simulink library "MBDS_Subsystems"  (R2018b)
settings: Solver=ode45  StartTime=0.0  StopTime=10.0  RelTol=1e-3
libraries: KIBES_Signal x1429, MBDS_Modules x44, simulink x2
(part 5 of 15)

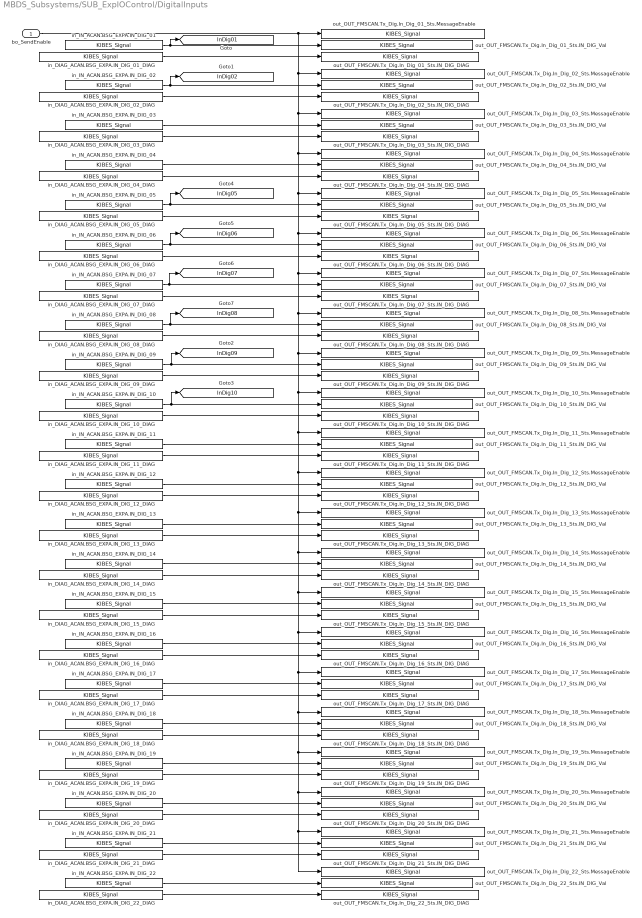
== system MBDS_Subsystems/SUB_ExpIOControl/DigitalInputs ==
  bo_SendEnable : Inport
  in_DIAG_ACAN.BSG_EXPA.IN_DIG_01_DIAG : KIBES_Signal/KIBES_Signal  MBDS_LibraryBlock=on  DatabaseKey=871  SignalName=DIAG_ACAN.BSG_EXPA.IN_DIG_01_DIAG  SymbolName=DIAG_ACAN_BSG_EXPA_IN_DIG_01_DIAG_000871  DataType=uint16  Init=1  Slope=1  Bias=0  DataSize=1  fpDataType=uint16  BlockIOType=Inport  DeviceType=0
  in_DIAG_ACAN.BSG_EXPA.IN_DIG_02_DIAG : KIBES_Signal/KIBES_Signal  MBDS_LibraryBlock=on  DatabaseKey=869  SignalName=DIAG_ACAN.BSG_EXPA.IN_DIG_02_DIAG  SymbolName=DIAG_ACAN_BSG_EXPA_IN_DIG_02_DIAG_000869  DataType=uint16  Init=1  Slope=1  Bias=0  DataSize=1  fpDataType=uint16  BlockIOType=Inport  DeviceType=0
  in_DIAG_ACAN.BSG_EXPA.IN_DIG_03_DIAG : KIBES_Signal/KIBES_Signal  MBDS_LibraryBlock=on  DatabaseKey=867  SignalName=DIAG_ACAN.BSG_EXPA.IN_DIG_03_DIAG  SymbolName=DIAG_ACAN_BSG_EXPA_IN_DIG_03_DIAG_000867  DataType=uint16  Init=1  Slope=1  Bias=0  DataSize=1  fpDataType=uint16  BlockIOType=Inport  DeviceType=0
  in_DIAG_ACAN.BSG_EXPA.IN_DIG_04_DIAG : KIBES_Signal/KIBES_Signal  MBDS_LibraryBlock=on  DatabaseKey=865  SignalName=DIAG_ACAN.BSG_EXPA.IN_DIG_04_DIAG  SymbolName=DIAG_ACAN_BSG_EXPA_IN_DIG_04_DIAG_000865  DataType=uint16  Init=1  Slope=1  Bias=0  DataSize=1  fpDataType=uint16  BlockIOType=Inport  DeviceType=0
  in_DIAG_ACAN.BSG_EXPA.IN_DIG_05_DIAG : KIBES_Signal/KIBES_Signal  MBDS_LibraryBlock=on  DatabaseKey=859  SignalName=DIAG_ACAN.BSG_EXPA.IN_DIG_05_DIAG  SymbolName=DIAG_ACAN_BSG_EXPA_IN_DIG_05_DIAG_000859  DataType=uint16  Init=1  Slope=1  Bias=0  DataSize=1  fpDataType=uint16  BlockIOType=Inport  DeviceType=0
  in_DIAG_ACAN.BSG_EXPA.IN_DIG_06_DIAG : KIBES_Signal/KIBES_Signal  MBDS_LibraryBlock=on  DatabaseKey=862  SignalName=DIAG_ACAN.BSG_EXPA.IN_DIG_06_DIAG  SymbolName=DIAG_ACAN_BSG_EXPA_IN_DIG_06_DIAG_000862  DataType=uint16  Init=1  Slope=1  Bias=0  DataSize=1  fpDataType=uint16  BlockIOType=Inport  DeviceType=0
  in_DIAG_ACAN.BSG_EXPA.IN_DIG_07_DIAG : KIBES_Signal/KIBES_Signal  MBDS_LibraryBlock=on  DatabaseKey=882  SignalName=DIAG_ACAN.BSG_EXPA.IN_DIG_07_DIAG  SymbolName=DIAG_ACAN_BSG_EXPA_IN_DIG_07_DIAG_000882  DataType=uint16  Init=1  Slope=1  Bias=0  DataSize=1  fpDataType=uint16  BlockIOType=Inport  DeviceType=0
  in_DIAG_ACAN.BSG_EXPA.IN_DIG_08_DIAG : KIBES_Signal/KIBES_Signal  MBDS_LibraryBlock=on  DatabaseKey=884  SignalName=DIAG_ACAN.BSG_EXPA.IN_DIG_08_DIAG  SymbolName=DIAG_ACAN_BSG_EXPA_IN_DIG_08_DIAG_000884  DataType=uint16  Init=1  Slope=1  Bias=0  DataSize=1  fpDataType=uint16  BlockIOType=Inport  DeviceType=0
  in_DIAG_ACAN.BSG_EXPA.IN_DIG_09_DIAG : KIBES_Signal/KIBES_Signal  MBDS_LibraryBlock=on  DatabaseKey=880  SignalName=DIAG_ACAN.BSG_EXPA.IN_DIG_09_DIAG  SymbolName=DIAG_ACAN_BSG_EXPA_IN_DIG_09_DIAG_000880  DataType=uint16  Init=1  Slope=1  Bias=0  DataSize=1  fpDataType=uint16  BlockIOType=Inport  DeviceType=0
  in_DIAG_ACAN.BSG_EXPA.IN_DIG_10_DIAG : KIBES_Signal/KIBES_Signal  MBDS_LibraryBlock=on  DatabaseKey=877  SignalName=DIAG_ACAN.BSG_EXPA.IN_DIG_10_DIAG  SymbolName=DIAG_ACAN_BSG_EXPA_IN_DIG_10_DIAG_000877  DataType=uint16  Init=1  Slope=1  Bias=0  DataSize=1  fpDataType=uint16  BlockIOType=Inport  DeviceType=0
  in_DIAG_ACAN.BSG_EXPA.IN_DIG_11_DIAG : KIBES_Signal/KIBES_Signal  MBDS_LibraryBlock=on  DatabaseKey=849  SignalName=DIAG_ACAN.BSG_EXPA.IN_DIG_11_DIAG  SymbolName=DIAG_ACAN_BSG_EXPA_IN_DIG_11_DIAG_000849  DataType=uint16  Init=1  Slope=1  Bias=0  DataSize=1  fpDataType=uint16  BlockIOType=Inport  DeviceType=0
  in_DIAG_ACAN.BSG_EXPA.IN_DIG_12_DIAG : KIBES_Signal/KIBES_Signal  MBDS_LibraryBlock=on  DatabaseKey=841  SignalName=DIAG_ACAN.BSG_EXPA.IN_DIG_12_DIAG  SymbolName=DIAG_ACAN_BSG_EXPA_IN_DIG_12_DIAG_000841  DataType=uint16  Init=1  Slope=1  Bias=0  DataSize=1  fpDataType=uint16  BlockIOType=Inport  DeviceType=0
  in_DIAG_ACAN.BSG_EXPA.IN_DIG_13_DIAG : KIBES_Signal/KIBES_Signal  MBDS_LibraryBlock=on  DatabaseKey=843  SignalName=DIAG_ACAN.BSG_EXPA.IN_DIG_13_DIAG  SymbolName=DIAG_ACAN_BSG_EXPA_IN_DIG_13_DIAG_000843  DataType=uint16  Init=1  Slope=1  Bias=0  DataSize=1  fpDataType=uint16  BlockIOType=Inport  DeviceType=0
  in_DIAG_ACAN.BSG_EXPA.IN_DIG_14_DIAG : KIBES_Signal/KIBES_Signal  MBDS_LibraryBlock=on  DatabaseKey=857  SignalName=DIAG_ACAN.BSG_EXPA.IN_DIG_14_DIAG  SymbolName=DIAG_ACAN_BSG_EXPA_IN_DIG_14_DIAG_000857  DataType=uint16  Init=1  Slope=1  Bias=0  DataSize=1  fpDataType=uint16  BlockIOType=Inport  DeviceType=0
  in_DIAG_ACAN.BSG_EXPA.IN_DIG_15_DIAG : KIBES_Signal/KIBES_Signal  MBDS_LibraryBlock=on  DatabaseKey=855  SignalName=DIAG_ACAN.BSG_EXPA.IN_DIG_15_DIAG  SymbolName=DIAG_ACAN_BSG_EXPA_IN_DIG_15_DIAG_000855  DataType=uint16  Init=1  Slope=1  Bias=0  DataSize=1  fpDataType=uint16  BlockIOType=Inport  DeviceType=0
  in_DIAG_ACAN.BSG_EXPA.IN_DIG_16_DIAG : KIBES_Signal/KIBES_Signal  MBDS_LibraryBlock=on  DatabaseKey=847  SignalName=DIAG_ACAN.BSG_EXPA.IN_DIG_16_DIAG  SymbolName=DIAG_ACAN_BSG_EXPA_IN_DIG_16_DIAG_000847  DataType=uint16  Init=1  Slope=1  Bias=0  DataSize=1  fpDataType=uint16  BlockIOType=Inport  DeviceType=0
  in_DIAG_ACAN.BSG_EXPA.IN_DIG_17_DIAG : KIBES_Signal/KIBES_Signal  MBDS_LibraryBlock=on  DatabaseKey=861  SignalName=DIAG_ACAN.BSG_EXPA.IN_DIG_17_DIAG  SymbolName=DIAG_ACAN_BSG_EXPA_IN_DIG_17_DIAG_000861  DataType=uint16  Init=1  Slope=1  Bias=0  DataSize=1  fpDataType=uint16  BlockIOType=Inport  DeviceType=0
  in_DIAG_ACAN.BSG_EXPA.IN_DIG_18_DIAG : KIBES_Signal/KIBES_Signal  MBDS_LibraryBlock=on  DatabaseKey=851  SignalName=DIAG_ACAN.BSG_EXPA.IN_DIG_18_DIAG  SymbolName=DIAG_ACAN_BSG_EXPA_IN_DIG_18_DIAG_000851  DataType=uint16  Init=1  Slope=1  Bias=0  DataSize=1  fpDataType=uint16  BlockIOType=Inport  DeviceType=0
  in_DIAG_ACAN.BSG_EXPA.IN_DIG_19_DIAG : KIBES_Signal/KIBES_Signal  MBDS_LibraryBlock=on  DatabaseKey=842  SignalName=DIAG_ACAN.BSG_EXPA.IN_DIG_19_DIAG  SymbolName=DIAG_ACAN_BSG_EXPA_IN_DIG_19_DIAG_000842  DataType=uint16  Init=1  Slope=1  Bias=0  DataSize=1  fpDataType=uint16  BlockIOType=Inport  DeviceType=0
  in_DIAG_ACAN.BSG_EXPA.IN_DIG_20_DIAG : KIBES_Signal/KIBES_Signal  MBDS_LibraryBlock=on  DatabaseKey=846  SignalName=DIAG_ACAN.BSG_EXPA.IN_DIG_20_DIAG  SymbolName=DIAG_ACAN_BSG_EXPA_IN_DIG_20_DIAG_000846  DataType=uint16  Init=1  Slope=1  Bias=0  DataSize=1  fpDataType=uint16  BlockIOType=Inport  DeviceType=0
  in_DIAG_ACAN.BSG_EXPA.IN_DIG_21_DIAG : KIBES_Signal/KIBES_Signal  MBDS_LibraryBlock=on  DatabaseKey=875  SignalName=DIAG_ACAN.BSG_EXPA.IN_DIG_21_DIAG  SymbolName=DIAG_ACAN_BSG_EXPA_IN_DIG_21_DIAG_000875  DataType=uint16  Init=1  Slope=1  Bias=0  DataSize=1  fpDataType=uint16  BlockIOType=Inport  DeviceType=0
  in_DIAG_ACAN.BSG_EXPA.IN_DIG_22_DIAG : KIBES_Signal/KIBES_Signal  MBDS_LibraryBlock=on  DatabaseKey=873  SignalName=DIAG_ACAN.BSG_EXPA.IN_DIG_22_DIAG  SymbolName=DIAG_ACAN_BSG_EXPA_IN_DIG_22_DIAG_000873  DataType=uint16  Init=1  Slope=1  Bias=0  DataSize=1  fpDataType=uint16  BlockIOType=Inport  DeviceType=0
  in_IN_ACAN.BSG_EXPA.IN_DIG_01 : KIBES_Signal/KIBES_Signal  MBDS_LibraryBlock=on  DatabaseKey=872  SignalName=IN_ACAN.BSG_EXPA.IN_DIG_01  SymbolName=IN_ACAN_BSG_EXPA_IN_DIG_01_000872  DataType=boolean  Init=0  Slope=1  Bias=0  DataSize=1  fpDataType=boolean  BlockIOType=Inport  DeviceType=0
  in_IN_ACAN.BSG_EXPA.IN_DIG_02 : KIBES_Signal/KIBES_Signal  MBDS_LibraryBlock=on  DatabaseKey=878  SignalName=IN_ACAN.BSG_EXPA.IN_DIG_02  SymbolName=IN_ACAN_BSG_EXPA_IN_DIG_02_000878  DataType=boolean  Init=0  Slope=1  Bias=0  DataSize=1  fpDataType=boolean  BlockIOType=Inport  DeviceType=0
  in_IN_ACAN.BSG_EXPA.IN_DIG_03 : KIBES_Signal/KIBES_Signal  MBDS_LibraryBlock=on  DatabaseKey=870  SignalName=IN_ACAN.BSG_EXPA.IN_DIG_03  SymbolName=IN_ACAN_BSG_EXPA_IN_DIG_03_000870  DataType=boolean  Init=0  Slope=1  Bias=0  DataSize=1  fpDataType=boolean  BlockIOType=Inport  DeviceType=0
  in_IN_ACAN.BSG_EXPA.IN_DIG_04 : KIBES_Signal/KIBES_Signal  MBDS_LibraryBlock=on  DatabaseKey=866  SignalName=IN_ACAN.BSG_EXPA.IN_DIG_04  SymbolName=IN_ACAN_BSG_EXPA_IN_DIG_04_000866  DataType=boolean  Init=0  Slope=1  Bias=0  DataSize=1  fpDataType=boolean  BlockIOType=Inport  DeviceType=0
  in_IN_ACAN.BSG_EXPA.IN_DIG_05 : KIBES_Signal/KIBES_Signal  MBDS_LibraryBlock=on  DatabaseKey=864  SignalName=IN_ACAN.BSG_EXPA.IN_DIG_05  SymbolName=IN_ACAN_BSG_EXPA_IN_DIG_05_000864  DataType=boolean  Init=0  Slope=1  Bias=0  DataSize=1  fpDataType=boolean  BlockIOType=Inport  DeviceType=0
  in_IN_ACAN.BSG_EXPA.IN_DIG_06 : KIBES_Signal/KIBES_Signal  MBDS_LibraryBlock=on  DatabaseKey=863  SignalName=IN_ACAN.BSG_EXPA.IN_DIG_06  SymbolName=IN_ACAN_BSG_EXPA_IN_DIG_06_000863  DataType=boolean  Init=0  Slope=1  Bias=0  DataSize=1  fpDataType=boolean  BlockIOType=Inport  DeviceType=0
  in_IN_ACAN.BSG_EXPA.IN_DIG_07 : KIBES_Signal/KIBES_Signal  MBDS_LibraryBlock=on  DatabaseKey=868  SignalName=IN_ACAN.BSG_EXPA.IN_DIG_07  SymbolName=IN_ACAN_BSG_EXPA_IN_DIG_07_000868  DataType=boolean  Init=0  Slope=1  Bias=0  DataSize=1  fpDataType=boolean  BlockIOType=Inport  DeviceType=0
  in_IN_ACAN.BSG_EXPA.IN_DIG_08 : KIBES_Signal/KIBES_Signal  MBDS_LibraryBlock=on  DatabaseKey=883  SignalName=IN_ACAN.BSG_EXPA.IN_DIG_08  SymbolName=IN_ACAN_BSG_EXPA_IN_DIG_08_000883  DataType=boolean  Init=0  Slope=1  Bias=0  DataSize=1  fpDataType=boolean  BlockIOType=Inport  DeviceType=0
  in_IN_ACAN.BSG_EXPA.IN_DIG_09 : KIBES_Signal/KIBES_Signal  MBDS_LibraryBlock=on  DatabaseKey=881  SignalName=IN_ACAN.BSG_EXPA.IN_DIG_09  SymbolName=IN_ACAN_BSG_EXPA_IN_DIG_09_000881  DataType=boolean  Init=0  Slope=1  Bias=0  DataSize=1  fpDataType=boolean  BlockIOType=Inport  DeviceType=0
  in_IN_ACAN.BSG_EXPA.IN_DIG_10 : KIBES_Signal/KIBES_Signal  MBDS_LibraryBlock=on  DatabaseKey=879  SignalName=IN_ACAN.BSG_EXPA.IN_DIG_10  SymbolName=IN_ACAN_BSG_EXPA_IN_DIG_10_000879  DataType=boolean  Init=0  Slope=1  Bias=0  DataSize=1  fpDataType=boolean  BlockIOType=Inport  DeviceType=0
  in_IN_ACAN.BSG_EXPA.IN_DIG_11 : KIBES_Signal/KIBES_Signal  MBDS_LibraryBlock=on  DatabaseKey=860  SignalName=IN_ACAN.BSG_EXPA.IN_DIG_11  SymbolName=IN_ACAN_BSG_EXPA_IN_DIG_11_000860  DataType=boolean  Init=0  Slope=1  Bias=0  DataSize=1  fpDataType=boolean  BlockIOType=Inport  DeviceType=0
  in_IN_ACAN.BSG_EXPA.IN_DIG_12 : KIBES_Signal/KIBES_Signal  MBDS_LibraryBlock=on  DatabaseKey=848  SignalName=IN_ACAN.BSG_EXPA.IN_DIG_12  SymbolName=IN_ACAN_BSG_EXPA_IN_DIG_12_000848  DataType=boolean  Init=0  Slope=1  Bias=0  DataSize=1  fpDataType=boolean  BlockIOType=Inport  DeviceType=0
  in_IN_ACAN.BSG_EXPA.IN_DIG_13 : KIBES_Signal/KIBES_Signal  MBDS_LibraryBlock=on  DatabaseKey=844  SignalName=IN_ACAN.BSG_EXPA.IN_DIG_13  SymbolName=IN_ACAN_BSG_EXPA_IN_DIG_13_000844  DataType=boolean  Init=0  Slope=1  Bias=0  DataSize=1  fpDataType=boolean  BlockIOType=Inport  DeviceType=0
  in_IN_ACAN.BSG_EXPA.IN_DIG_14 : KIBES_Signal/KIBES_Signal  MBDS_LibraryBlock=on  DatabaseKey=858  SignalName=IN_ACAN.BSG_EXPA.IN_DIG_14  SymbolName=IN_ACAN_BSG_EXPA_IN_DIG_14_000858  DataType=boolean  Init=0  Slope=1  Bias=0  DataSize=1  fpDataType=boolean  BlockIOType=Inport  DeviceType=0
  in_IN_ACAN.BSG_EXPA.IN_DIG_15 : KIBES_Signal/KIBES_Signal  MBDS_LibraryBlock=on  DatabaseKey=856  SignalName=IN_ACAN.BSG_EXPA.IN_DIG_15  SymbolName=IN_ACAN_BSG_EXPA_IN_DIG_15_000856  DataType=boolean  Init=0  Slope=1  Bias=0  DataSize=1  fpDataType=boolean  BlockIOType=Inport  DeviceType=0
  in_IN_ACAN.BSG_EXPA.IN_DIG_16 : KIBES_Signal/KIBES_Signal  MBDS_LibraryBlock=on  DatabaseKey=854  SignalName=IN_ACAN.BSG_EXPA.IN_DIG_16  SymbolName=IN_ACAN_BSG_EXPA_IN_DIG_16_000854  DataType=boolean  Init=0  Slope=1  Bias=0  DataSize=1  fpDataType=boolean  BlockIOType=Inport  DeviceType=0
  in_IN_ACAN.BSG_EXPA.IN_DIG_17 : KIBES_Signal/KIBES_Signal  MBDS_LibraryBlock=on  DatabaseKey=853  SignalName=IN_ACAN.BSG_EXPA.IN_DIG_17  SymbolName=IN_ACAN_BSG_EXPA_IN_DIG_17_000853  DataType=boolean  Init=0  Slope=1  Bias=0  DataSize=1  fpDataType=boolean  BlockIOType=Inport  DeviceType=0
  in_IN_ACAN.BSG_EXPA.IN_DIG_18 : KIBES_Signal/KIBES_Signal  MBDS_LibraryBlock=on  DatabaseKey=852  SignalName=IN_ACAN.BSG_EXPA.IN_DIG_18  SymbolName=IN_ACAN_BSG_EXPA_IN_DIG_18_000852  DataType=boolean  Init=0  Slope=1  Bias=0  DataSize=1  fpDataType=boolean  BlockIOType=Inport  DeviceType=0
  in_IN_ACAN.BSG_EXPA.IN_DIG_19 : KIBES_Signal/KIBES_Signal  MBDS_LibraryBlock=on  DatabaseKey=845  SignalName=IN_ACAN.BSG_EXPA.IN_DIG_19  SymbolName=IN_ACAN_BSG_EXPA_IN_DIG_19_000845  DataType=boolean  Init=0  Slope=1  Bias=0  DataSize=1  fpDataType=boolean  BlockIOType=Inport  DeviceType=0
  in_IN_ACAN.BSG_EXPA.IN_DIG_20 : KIBES_Signal/KIBES_Signal  MBDS_LibraryBlock=on  DatabaseKey=850  SignalName=IN_ACAN.BSG_EXPA.IN_DIG_20  SymbolName=IN_ACAN_BSG_EXPA_IN_DIG_20_000850  DataType=boolean  Init=0  Slope=1  Bias=0  DataSize=1  fpDataType=boolean  BlockIOType=Inport  DeviceType=0
  in_IN_ACAN.BSG_EXPA.IN_DIG_21 : KIBES_Signal/KIBES_Signal  MBDS_LibraryBlock=on  DatabaseKey=876  SignalName=IN_ACAN.BSG_EXPA.IN_DIG_21  SymbolName=IN_ACAN_BSG_EXPA_IN_DIG_21_000876  DataType=boolean  Init=0  Slope=1  Bias=0  DataSize=1  fpDataType=boolean  BlockIOType=Inport  DeviceType=0
  in_IN_ACAN.BSG_EXPA.IN_DIG_22 : KIBES_Signal/KIBES_Signal  MBDS_LibraryBlock=on  DatabaseKey=874  SignalName=IN_ACAN.BSG_EXPA.IN_DIG_22  SymbolName=IN_ACAN_BSG_EXPA_IN_DIG_22_000874  DataType=boolean  Init=0  Slope=1  Bias=0  DataSize=1  fpDataType=boolean  BlockIOType=Inport  DeviceType=0
  out_OUT_FMSCAN.Tx_Dig.In_Dig_01_Sts.IN_DIG_DIAG : KIBES_Signal/KIBES_Signal  MBDS_LibraryBlock=on  DatabaseKey=2366  SignalName=OUT_FMSCAN.Tx_Dig.In_Dig_01_Sts.IN_DIG_DIAG  SymbolName=OUT_FMSCAN_Tx_Dig_In_Dig_01_Sts_IN_DIG_DIAG_002366  DataType=uint16  Init=0  Slope=1  Bias=0  DataSize=1  fpDataType=uint16  BlockIOType=Outport  DeviceType=0
  out_OUT_FMSCAN.Tx_Dig.In_Dig_01_Sts.IN_DIG_Val : KIBES_Signal/KIBES_Signal  MBDS_LibraryBlock=on  DatabaseKey=2367  SignalName=OUT_FMSCAN.Tx_Dig.In_Dig_01_Sts.IN_DIG_Val  SymbolName=OUT_FMSCAN_Tx_Dig_In_Dig_01_Sts_IN_DIG_Val_002367  DataType=boolean  Init=0  Slope=1  Bias=0  DataSize=1  fpDataType=boolean  BlockIOType=Outport  DeviceType=0
  out_OUT_FMSCAN.Tx_Dig.In_Dig_01_Sts.MessageEnable : KIBES_Signal/KIBES_Signal  MBDS_LibraryBlock=on  DatabaseKey=2410  SignalName=OUT_FMSCAN.Tx_Dig.In_Dig_01_Sts.MessageEnable  SymbolName=OUT_FMSCAN_Tx_Dig_In_Dig_01_Sts_MessageEnable_002410  DataType=boolean  Init=0  Slope=1  Bias=0  DataSize=1  fpDataType=boolean  BlockIOType=Outport  DeviceType=0
  out_OUT_FMSCAN.Tx_Dig.In_Dig_02_Sts.IN_DIG_DIAG : KIBES_Signal/KIBES_Signal  MBDS_LibraryBlock=on  DatabaseKey=2368  SignalName=OUT_FMSCAN.Tx_Dig.In_Dig_02_Sts.IN_DIG_DIAG  SymbolName=OUT_FMSCAN_Tx_Dig_In_Dig_02_Sts_IN_DIG_DIAG_002368  DataType=uint16  Init=0  Slope=1  Bias=0  DataSize=1  fpDataType=uint16  BlockIOType=Outport  DeviceType=0
  out_OUT_FMSCAN.Tx_Dig.In_Dig_02_Sts.IN_DIG_Val : KIBES_Signal/KIBES_Signal  MBDS_LibraryBlock=on  DatabaseKey=2369  SignalName=OUT_FMSCAN.Tx_Dig.In_Dig_02_Sts.IN_DIG_Val  SymbolName=OUT_FMSCAN_Tx_Dig_In_Dig_02_Sts_IN_DIG_Val_002369  DataType=boolean  Init=0  Slope=1  Bias=0  DataSize=1  fpDataType=boolean  BlockIOType=Outport  DeviceType=0
  out_OUT_FMSCAN.Tx_Dig.In_Dig_02_Sts.MessageEnable : KIBES_Signal/KIBES_Signal  MBDS_LibraryBlock=on  DatabaseKey=2411  SignalName=OUT_FMSCAN.Tx_Dig.In_Dig_02_Sts.MessageEnable  SymbolName=OUT_FMSCAN_Tx_Dig_In_Dig_02_Sts_MessageEnable_002411  DataType=boolean  Init=0  Slope=1  Bias=0  DataSize=1  fpDataType=boolean  BlockIOType=Outport  DeviceType=0
  out_OUT_FMSCAN.Tx_Dig.In_Dig_03_Sts.IN_DIG_DIAG : KIBES_Signal/KIBES_Signal  MBDS_LibraryBlock=on  DatabaseKey=2370  SignalName=OUT_FMSCAN.Tx_Dig.In_Dig_03_Sts.IN_DIG_DIAG  SymbolName=OUT_FMSCAN_Tx_Dig_In_Dig_03_Sts_IN_DIG_DIAG_002370  DataType=uint16  Init=0  Slope=1  Bias=0  DataSize=1  fpDataType=uint16  BlockIOType=Outport  DeviceType=0
  out_OUT_FMSCAN.Tx_Dig.In_Dig_03_Sts.IN_DIG_Val : KIBES_Signal/KIBES_Signal  MBDS_LibraryBlock=on  DatabaseKey=2371  SignalName=OUT_FMSCAN.Tx_Dig.In_Dig_03_Sts.IN_DIG_Val  SymbolName=OUT_FMSCAN_Tx_Dig_In_Dig_03_Sts_IN_DIG_Val_002371  DataType=boolean  Init=0  Slope=1  Bias=0  DataSize=1  fpDataType=boolean  BlockIOType=Outport  DeviceType=0
  out_OUT_FMSCAN.Tx_Dig.In_Dig_03_Sts.MessageEnable : KIBES_Signal/KIBES_Signal  MBDS_LibraryBlock=on  DatabaseKey=2412  SignalName=OUT_FMSCAN.Tx_Dig.In_Dig_03_Sts.MessageEnable  SymbolName=OUT_FMSCAN_Tx_Dig_In_Dig_03_Sts_MessageEnable_002412  DataType=boolean  Init=0  Slope=1  Bias=0  DataSize=1  fpDataType=boolean  BlockIOType=Outport  DeviceType=0
  out_OUT_FMSCAN.Tx_Dig.In_Dig_04_Sts.IN_DIG_DIAG : KIBES_Signal/KIBES_Signal  MBDS_LibraryBlock=on  DatabaseKey=2372  SignalName=OUT_FMSCAN.Tx_Dig.In_Dig_04_Sts.IN_DIG_DIAG  SymbolName=OUT_FMSCAN_Tx_Dig_In_Dig_04_Sts_IN_DIG_DIAG_002372  DataType=uint16  Init=0  Slope=1  Bias=0  DataSize=1  fpDataType=uint16  BlockIOType=Outport  DeviceType=0
  out_OUT_FMSCAN.Tx_Dig.In_Dig_04_Sts.IN_DIG_Val : KIBES_Signal/KIBES_Signal  MBDS_LibraryBlock=on  DatabaseKey=2373  SignalName=OUT_FMSCAN.Tx_Dig.In_Dig_04_Sts.IN_DIG_Val  SymbolName=OUT_FMSCAN_Tx_Dig_In_Dig_04_Sts_IN_DIG_Val_002373  DataType=boolean  Init=0  Slope=1  Bias=0  DataSize=1  fpDataType=boolean  BlockIOType=Outport  DeviceType=0
  out_OUT_FMSCAN.Tx_Dig.In_Dig_04_Sts.MessageEnable : KIBES_Signal/KIBES_Signal  MBDS_LibraryBlock=on  DatabaseKey=2413  SignalName=OUT_FMSCAN.Tx_Dig.In_Dig_04_Sts.MessageEnable  SymbolName=OUT_FMSCAN_Tx_Dig_In_Dig_04_Sts_MessageEnable_002413  DataType=boolean  Init=0  Slope=1  Bias=0  DataSize=1  fpDataType=boolean  BlockIOType=Outport  DeviceType=0
  out_OUT_FMSCAN.Tx_Dig.In_Dig_05_Sts.IN_DIG_DIAG : KIBES_Signal/KIBES_Signal  MBDS_LibraryBlock=on  DatabaseKey=2374  SignalName=OUT_FMSCAN.Tx_Dig.In_Dig_05_Sts.IN_DIG_DIAG  SymbolName=OUT_FMSCAN_Tx_Dig_In_Dig_05_Sts_IN_DIG_DIAG_002374  DataType=uint16  Init=0  Slope=1  Bias=0  DataSize=1  fpDataType=uint16  BlockIOType=Outport  DeviceType=0
  out_OUT_FMSCAN.Tx_Dig.In_Dig_05_Sts.IN_DIG_Val : KIBES_Signal/KIBES_Signal  MBDS_LibraryBlock=on  DatabaseKey=2375  SignalName=OUT_FMSCAN.Tx_Dig.In_Dig_05_Sts.IN_DIG_Val  SymbolName=OUT_FMSCAN_Tx_Dig_In_Dig_05_Sts_IN_DIG_Val_002375  DataType=boolean  Init=0  Slope=1  Bias=0  DataSize=1  fpDataType=boolean  BlockIOType=Outport  DeviceType=0
  out_OUT_FMSCAN.Tx_Dig.In_Dig_05_Sts.MessageEnable : KIBES_Signal/KIBES_Signal  MBDS_LibraryBlock=on  DatabaseKey=2414  SignalName=OUT_FMSCAN.Tx_Dig.In_Dig_05_Sts.MessageEnable  SymbolName=OUT_FMSCAN_Tx_Dig_In_Dig_05_Sts_MessageEnable_002414  DataType=boolean  Init=0  Slope=1  Bias=0  DataSize=1  fpDataType=boolean  BlockIOType=Outport  DeviceType=0
  out_OUT_FMSCAN.Tx_Dig.In_Dig_06_Sts.IN_DIG_DIAG : KIBES_Signal/KIBES_Signal  MBDS_LibraryBlock=on  DatabaseKey=2376  SignalName=OUT_FMSCAN.Tx_Dig.In_Dig_06_Sts.IN_DIG_DIAG  SymbolName=OUT_FMSCAN_Tx_Dig_In_Dig_06_Sts_IN_DIG_DIAG_002376  DataType=uint16  Init=0  Slope=1  Bias=0  DataSize=1  fpDataType=uint16  BlockIOType=Outport  DeviceType=0
  out_OUT_FMSCAN.Tx_Dig.In_Dig_06_Sts.IN_DIG_Val : KIBES_Signal/KIBES_Signal  MBDS_LibraryBlock=on  DatabaseKey=2377  SignalName=OUT_FMSCAN.Tx_Dig.In_Dig_06_Sts.IN_DIG_Val  SymbolName=OUT_FMSCAN_Tx_Dig_In_Dig_06_Sts_IN_DIG_Val_002377  DataType=boolean  Init=0  Slope=1  Bias=0  DataSize=1  fpDataType=boolean  BlockIOType=Outport  DeviceType=0
  out_OUT_FMSCAN.Tx_Dig.In_Dig_06_Sts.MessageEnable : KIBES_Signal/KIBES_Signal  MBDS_LibraryBlock=on  DatabaseKey=2415  SignalName=OUT_FMSCAN.Tx_Dig.In_Dig_06_Sts.MessageEnable  SymbolName=OUT_FMSCAN_Tx_Dig_In_Dig_06_Sts_MessageEnable_002415  DataType=boolean  Init=0  Slope=1  Bias=0  DataSize=1  fpDataType=boolean  BlockIOType=Outport  DeviceType=0
  out_OUT_FMSCAN.Tx_Dig.In_Dig_07_Sts.IN_DIG_DIAG : KIBES_Signal/KIBES_Signal  MBDS_LibraryBlock=on  DatabaseKey=2378  SignalName=OUT_FMSCAN.Tx_Dig.In_Dig_07_Sts.IN_DIG_DIAG  SymbolName=OUT_FMSCAN_Tx_Dig_In_Dig_07_Sts_IN_DIG_DIAG_002378  DataType=uint16  Init=0  Slope=1  Bias=0  DataSize=1  fpDataType=uint16  BlockIOType=Outport  DeviceType=0
  out_OUT_FMSCAN.Tx_Dig.In_Dig_07_Sts.IN_DIG_Val : KIBES_Signal/KIBES_Signal  MBDS_LibraryBlock=on  DatabaseKey=2379  SignalName=OUT_FMSCAN.Tx_Dig.In_Dig_07_Sts.IN_DIG_Val  SymbolName=OUT_FMSCAN_Tx_Dig_In_Dig_07_Sts_IN_DIG_Val_002379  DataType=boolean  Init=0  Slope=1  Bias=0  DataSize=1  fpDataType=boolean  BlockIOType=Outport  DeviceType=0
  out_OUT_FMSCAN.Tx_Dig.In_Dig_07_Sts.MessageEnable : KIBES_Signal/KIBES_Signal  MBDS_LibraryBlock=on  DatabaseKey=2416  SignalName=OUT_FMSCAN.Tx_Dig.In_Dig_07_Sts.MessageEnable  SymbolName=OUT_FMSCAN_Tx_Dig_In_Dig_07_Sts_MessageEnable_002416  DataType=boolean  Init=0  Slope=1  Bias=0  DataSize=1  fpDataType=boolean  BlockIOType=Outport  DeviceType=0
  out_OUT_FMSCAN.Tx_Dig.In_Dig_08_Sts.IN_DIG_DIAG : KIBES_Signal/KIBES_Signal  MBDS_LibraryBlock=on  DatabaseKey=2380  SignalName=OUT_FMSCAN.Tx_Dig.In_Dig_08_Sts.IN_DIG_DIAG  SymbolName=OUT_FMSCAN_Tx_Dig_In_Dig_08_Sts_IN_DIG_DIAG_002380  DataType=uint16  Init=0  Slope=1  Bias=0  DataSize=1  fpDataType=uint16  BlockIOType=Outport  DeviceType=0
  out_OUT_FMSCAN.Tx_Dig.In_Dig_08_Sts.IN_DIG_Val : KIBES_Signal/KIBES_Signal  MBDS_LibraryBlock=on  DatabaseKey=2381  SignalName=OUT_FMSCAN.Tx_Dig.In_Dig_08_Sts.IN_DIG_Val  SymbolName=OUT_FMSCAN_Tx_Dig_In_Dig_08_Sts_IN_DIG_Val_002381  DataType=boolean  Init=0  Slope=1  Bias=0  DataSize=1  fpDataType=boolean  BlockIOType=Outport  DeviceType=0
  out_OUT_FMSCAN.Tx_Dig.In_Dig_08_Sts.MessageEnable : KIBES_Signal/KIBES_Signal  MBDS_LibraryBlock=on  DatabaseKey=2417  SignalName=OUT_FMSCAN.Tx_Dig.In_Dig_08_Sts.MessageEnable  SymbolName=OUT_FMSCAN_Tx_Dig_In_Dig_08_Sts_MessageEnable_002417  DataType=boolean  Init=0  Slope=1  Bias=0  DataSize=1  fpDataType=boolean  BlockIOType=Outport  DeviceType=0
  out_OUT_FMSCAN.Tx_Dig.In_Dig_09_Sts.IN_DIG_DIAG : KIBES_Signal/KIBES_Signal  MBDS_LibraryBlock=on  DatabaseKey=2382  SignalName=OUT_FMSCAN.Tx_Dig.In_Dig_09_Sts.IN_DIG_DIAG  SymbolName=OUT_FMSCAN_Tx_Dig_In_Dig_09_Sts_IN_DIG_DIAG_002382  DataType=uint16  Init=0  Slope=1  Bias=0  DataSize=1  fpDataType=uint16  BlockIOType=Outport  DeviceType=0
  out_OUT_FMSCAN.Tx_Dig.In_Dig_09_Sts.IN_DIG_Val : KIBES_Signal/KIBES_Signal  MBDS_LibraryBlock=on  DatabaseKey=2383  SignalName=OUT_FMSCAN.Tx_Dig.In_Dig_09_Sts.IN_DIG_Val  SymbolName=OUT_FMSCAN_Tx_Dig_In_Dig_09_Sts_IN_DIG_Val_002383  DataType=boolean  Init=0  Slope=1  Bias=0  DataSize=1  fpDataType=boolean  BlockIOType=Outport  DeviceType=0
  out_OUT_FMSCAN.Tx_Dig.In_Dig_09_Sts.MessageEnable : KIBES_Signal/KIBES_Signal  MBDS_LibraryBlock=on  DatabaseKey=2418  SignalName=OUT_FMSCAN.Tx_Dig.In_Dig_09_Sts.MessageEnable  SymbolName=OUT_FMSCAN_Tx_Dig_In_Dig_09_Sts_MessageEnable_002418  DataType=boolean  Init=0  Slope=1  Bias=0  DataSize=1  fpDataType=boolean  BlockIOType=Outport  DeviceType=0
  out_OUT_FMSCAN.Tx_Dig.In_Dig_10_Sts.IN_DIG_DIAG : KIBES_Signal/KIBES_Signal  MBDS_LibraryBlock=on  DatabaseKey=2384  SignalName=OUT_FMSCAN.Tx_Dig.In_Dig_10_Sts.IN_DIG_DIAG  SymbolName=OUT_FMSCAN_Tx_Dig_In_Dig_10_Sts_IN_DIG_DIAG_002384  DataType=uint16  Init=0  Slope=1  Bias=0  DataSize=1  fpDataType=uint16  BlockIOType=Outport  DeviceType=0
  out_OUT_FMSCAN.Tx_Dig.In_Dig_10_Sts.IN_DIG_Val : KIBES_Signal/KIBES_Signal  MBDS_LibraryBlock=on  DatabaseKey=2385  SignalName=OUT_FMSCAN.Tx_Dig.In_Dig_10_Sts.IN_DIG_Val  SymbolName=OUT_FMSCAN_Tx_Dig_In_Dig_10_Sts_IN_DIG_Val_002385  DataType=boolean  Init=0  Slope=1  Bias=0  DataSize=1  fpDataType=boolean  BlockIOType=Outport  DeviceType=0
  out_OUT_FMSCAN.Tx_Dig.In_Dig_10_Sts.MessageEnable : KIBES_Signal/KIBES_Signal  MBDS_LibraryBlock=on  DatabaseKey=2419  SignalName=OUT_FMSCAN.Tx_Dig.In_Dig_10_Sts.MessageEnable  SymbolName=OUT_FMSCAN_Tx_Dig_In_Dig_10_Sts_MessageEnable_002419  DataType=boolean  Init=0  Slope=1  Bias=0  DataSize=1  fpDataType=boolean  BlockIOType=Outport  DeviceType=0
  out_OUT_FMSCAN.Tx_Dig.In_Dig_11_Sts.IN_DIG_DIAG : KIBES_Signal/KIBES_Signal  MBDS_LibraryBlock=on  DatabaseKey=2386  SignalName=OUT_FMSCAN.Tx_Dig.In_Dig_11_Sts.IN_DIG_DIAG  SymbolName=OUT_FMSCAN_Tx_Dig_In_Dig_11_Sts_IN_DIG_DIAG_002386  DataType=uint16  Init=0  Slope=1  Bias=0  DataSize=1  fpDataType=uint16  BlockIOType=Outport  DeviceType=0
  out_OUT_FMSCAN.Tx_Dig.In_Dig_11_Sts.IN_DIG_Val : KIBES_Signal/KIBES_Signal  MBDS_LibraryBlock=on  DatabaseKey=2387  SignalName=OUT_FMSCAN.Tx_Dig.In_Dig_11_Sts.IN_DIG_Val  SymbolName=OUT_FMSCAN_Tx_Dig_In_Dig_11_Sts_IN_DIG_Val_002387  DataType=boolean  Init=0  Slope=1  Bias=0  DataSize=1  fpDataType=boolean  BlockIOType=Outport  DeviceType=0
  out_OUT_FMSCAN.Tx_Dig.In_Dig_11_Sts.MessageEnable : KIBES_Signal/KIBES_Signal  MBDS_LibraryBlock=on  DatabaseKey=2420  SignalName=OUT_FMSCAN.Tx_Dig.In_Dig_11_Sts.MessageEnable  SymbolName=OUT_FMSCAN_Tx_Dig_In_Dig_11_Sts_MessageEnable_002420  DataType=boolean  Init=0  Slope=1  Bias=0  DataSize=1  fpDataType=boolean  BlockIOType=Outport  DeviceType=0
  out_OUT_FMSCAN.Tx_Dig.In_Dig_12_Sts.IN_DIG_DIAG : KIBES_Signal/KIBES_Signal  MBDS_LibraryBlock=on  DatabaseKey=2388  SignalName=OUT_FMSCAN.Tx_Dig.In_Dig_12_Sts.IN_DIG_DIAG  SymbolName=OUT_FMSCAN_Tx_Dig_In_Dig_12_Sts_IN_DIG_DIAG_002388  DataType=uint16  Init=0  Slope=1  Bias=0  DataSize=1  fpDataType=uint16  BlockIOType=Outport  DeviceType=0
  out_OUT_FMSCAN.Tx_Dig.In_Dig_12_Sts.IN_DIG_Val : KIBES_Signal/KIBES_Signal  MBDS_LibraryBlock=on  DatabaseKey=2389  SignalName=OUT_FMSCAN.Tx_Dig.In_Dig_12_Sts.IN_DIG_Val  SymbolName=OUT_FMSCAN_Tx_Dig_In_Dig_12_Sts_IN_DIG_Val_002389  DataType=boolean  Init=0  Slope=1  Bias=0  DataSize=1  fpDataType=boolean  BlockIOType=Outport  DeviceType=0
  out_OUT_FMSCAN.Tx_Dig.In_Dig_12_Sts.MessageEnable : KIBES_Signal/KIBES_Signal  MBDS_LibraryBlock=on  DatabaseKey=2421  SignalName=OUT_FMSCAN.Tx_Dig.In_Dig_12_Sts.MessageEnable  SymbolName=OUT_FMSCAN_Tx_Dig_In_Dig_12_Sts_MessageEnable_002421  DataType=boolean  Init=0  Slope=1  Bias=0  DataSize=1  fpDataType=boolean  BlockIOType=Outport  DeviceType=0
  out_OUT_FMSCAN.Tx_Dig.In_Dig_13_Sts.IN_DIG_DIAG : KIBES_Signal/KIBES_Signal  MBDS_LibraryBlock=on  DatabaseKey=2390  SignalName=OUT_FMSCAN.Tx_Dig.In_Dig_13_Sts.IN_DIG_DIAG  SymbolName=OUT_FMSCAN_Tx_Dig_In_Dig_13_Sts_IN_DIG_DIAG_002390  DataType=uint16  Init=0  Slope=1  Bias=0  DataSize=1  fpDataType=uint16  BlockIOType=Outport  DeviceType=0
  out_OUT_FMSCAN.Tx_Dig.In_Dig_13_Sts.IN_DIG_Val : KIBES_Signal/KIBES_Signal  MBDS_LibraryBlock=on  DatabaseKey=2391  SignalName=OUT_FMSCAN.Tx_Dig.In_Dig_13_Sts.IN_DIG_Val  SymbolName=OUT_FMSCAN_Tx_Dig_In_Dig_13_Sts_IN_DIG_Val_002391  DataType=boolean  Init=0  Slope=1  Bias=0  DataSize=1  fpDataType=boolean  BlockIOType=Outport  DeviceType=0
  out_OUT_FMSCAN.Tx_Dig.In_Dig_13_Sts.MessageEnable : KIBES_Signal/KIBES_Signal  MBDS_LibraryBlock=on  DatabaseKey=2422  SignalName=OUT_FMSCAN.Tx_Dig.In_Dig_13_Sts.MessageEnable  SymbolName=OUT_FMSCAN_Tx_Dig_In_Dig_13_Sts_MessageEnable_002422  DataType=boolean  Init=0  Slope=1  Bias=0  DataSize=1  fpDataType=boolean  BlockIOType=Outport  DeviceType=0
  out_OUT_FMSCAN.Tx_Dig.In_Dig_14_Sts.IN_DIG_DIAG : KIBES_Signal/KIBES_Signal  MBDS_LibraryBlock=on  DatabaseKey=2392  SignalName=OUT_FMSCAN.Tx_Dig.In_Dig_14_Sts.IN_DIG_DIAG  SymbolName=OUT_FMSCAN_Tx_Dig_In_Dig_14_Sts_IN_DIG_DIAG_002392  DataType=uint16  Init=0  Slope=1  Bias=0  DataSize=1  fpDataType=uint16  BlockIOType=Outport  DeviceType=0
  out_OUT_FMSCAN.Tx_Dig.In_Dig_14_Sts.IN_DIG_Val : KIBES_Signal/KIBES_Signal  MBDS_LibraryBlock=on  DatabaseKey=2393  SignalName=OUT_FMSCAN.Tx_Dig.In_Dig_14_Sts.IN_DIG_Val  SymbolName=OUT_FMSCAN_Tx_Dig_In_Dig_14_Sts_IN_DIG_Val_002393  DataType=boolean  Init=0  Slope=1  Bias=0  DataSize=1  fpDataType=boolean  BlockIOType=Outport  DeviceType=0
  out_OUT_FMSCAN.Tx_Dig.In_Dig_14_Sts.MessageEnable : KIBES_Signal/KIBES_Signal  MBDS_LibraryBlock=on  DatabaseKey=2423  SignalName=OUT_FMSCAN.Tx_Dig.In_Dig_14_Sts.MessageEnable  SymbolName=OUT_FMSCAN_Tx_Dig_In_Dig_14_Sts_MessageEnable_002423  DataType=boolean  Init=0  Slope=1  Bias=0  DataSize=1  fpDataType=boolean  BlockIOType=Outport  DeviceType=0
  out_OUT_FMSCAN.Tx_Dig.In_Dig_15_Sts.IN_DIG_DIAG : KIBES_Signal/KIBES_Signal  MBDS_LibraryBlock=on  DatabaseKey=2394  SignalName=OUT_FMSCAN.Tx_Dig.In_Dig_15_Sts.IN_DIG_DIAG  SymbolName=OUT_FMSCAN_Tx_Dig_In_Dig_15_Sts_IN_DIG_DIAG_002394  DataType=uint16  Init=0  Slope=1  Bias=0  DataSize=1  fpDataType=uint16  BlockIOType=Outport  DeviceType=0
  out_OUT_FMSCAN.Tx_Dig.In_Dig_15_Sts.IN_DIG_Val : KIBES_Signal/KIBES_Signal  MBDS_LibraryBlock=on  DatabaseKey=2395  SignalName=OUT_FMSCAN.Tx_Dig.In_Dig_15_Sts.IN_DIG_Val  SymbolName=OUT_FMSCAN_Tx_Dig_In_Dig_15_Sts_IN_DIG_Val_002395  DataType=boolean  Init=0  Slope=1  Bias=0  DataSize=1  fpDataType=boolean  BlockIOType=Outport  DeviceType=0
  out_OUT_FMSCAN.Tx_Dig.In_Dig_15_Sts.MessageEnable : KIBES_Signal/KIBES_Signal  MBDS_LibraryBlock=on  DatabaseKey=2424  SignalName=OUT_FMSCAN.Tx_Dig.In_Dig_15_Sts.MessageEnable  SymbolName=OUT_FMSCAN_Tx_Dig_In_Dig_15_Sts_MessageEnable_002424  DataType=boolean  Init=0  Slope=1  Bias=0  DataSize=1  fpDataType=boolean  BlockIOType=Outport  DeviceType=0
  out_OUT_FMSCAN.Tx_Dig.In_Dig_16_Sts.IN_DIG_DIAG : KIBES_Signal/KIBES_Signal  MBDS_LibraryBlock=on  DatabaseKey=2396  SignalName=OUT_FMSCAN.Tx_Dig.In_Dig_16_Sts.IN_DIG_DIAG  SymbolName=OUT_FMSCAN_Tx_Dig_In_Dig_16_Sts_IN_DIG_DIAG_002396  DataType=uint16  Init=0  Slope=1  Bias=0  DataSize=1  fpDataType=uint16  BlockIOType=Outport  DeviceType=0
  out_OUT_FMSCAN.Tx_Dig.In_Dig_16_Sts.IN_DIG_Val : KIBES_Signal/KIBES_Signal  MBDS_LibraryBlock=on  DatabaseKey=2397  SignalName=OUT_FMSCAN.Tx_Dig.In_Dig_16_Sts.IN_DIG_Val  SymbolName=OUT_FMSCAN_Tx_Dig_In_Dig_16_Sts_IN_DIG_Val_002397  DataType=boolean  Init=0  Slope=1  Bias=0  DataSize=1  fpDataType=boolean  BlockIOType=Outport  DeviceType=0
  out_OUT_FMSCAN.Tx_Dig.In_Dig_16_Sts.MessageEnable : KIBES_Signal/KIBES_Signal  MBDS_LibraryBlock=on  DatabaseKey=2425  SignalName=OUT_FMSCAN.Tx_Dig.In_Dig_16_Sts.MessageEnable  SymbolName=OUT_FMSCAN_Tx_Dig_In_Dig_16_Sts_MessageEnable_002425  DataType=boolean  Init=0  Slope=1  Bias=0  DataSize=1  fpDataType=boolean  BlockIOType=Outport  DeviceType=0
  out_OUT_FMSCAN.Tx_Dig.In_Dig_17_Sts.IN_DIG_DIAG : KIBES_Signal/KIBES_Signal  MBDS_LibraryBlock=on  DatabaseKey=2398  SignalName=OUT_FMSCAN.Tx_Dig.In_Dig_17_Sts.IN_DIG_DIAG  SymbolName=OUT_FMSCAN_Tx_Dig_In_Dig_17_Sts_IN_DIG_DIAG_002398  DataType=uint16  Init=0  Slope=1  Bias=0  DataSize=1  fpDataType=uint16  BlockIOType=Outport  DeviceType=0
  out_OUT_FMSCAN.Tx_Dig.In_Dig_17_Sts.IN_DIG_Val : KIBES_Signal/KIBES_Signal  MBDS_LibraryBlock=on  DatabaseKey=2399  SignalName=OUT_FMSCAN.Tx_Dig.In_Dig_17_Sts.IN_DIG_Val  SymbolName=OUT_FMSCAN_Tx_Dig_In_Dig_17_Sts_IN_DIG_Val_002399  DataType=boolean  Init=0  Slope=1  Bias=0  DataSize=1  fpDataType=boolean  BlockIOType=Outport  DeviceType=0
  out_OUT_FMSCAN.Tx_Dig.In_Dig_17_Sts.MessageEnable : KIBES_Signal/KIBES_Signal  MBDS_LibraryBlock=on  DatabaseKey=2426  SignalName=OUT_FMSCAN.Tx_Dig.In_Dig_17_Sts.MessageEnable  SymbolName=OUT_FMSCAN_Tx_Dig_In_Dig_17_Sts_MessageEnable_002426  DataType=boolean  Init=0  Slope=1  Bias=0  DataSize=1  fpDataType=boolean  BlockIOType=Outport  DeviceType=0
  out_OUT_FMSCAN.Tx_Dig.In_Dig_18_Sts.IN_DIG_DIAG : KIBES_Signal/KIBES_Signal  MBDS_LibraryBlock=on  DatabaseKey=2400  SignalName=OUT_FMSCAN.Tx_Dig.In_Dig_18_Sts.IN_DIG_DIAG  SymbolName=OUT_FMSCAN_Tx_Dig_In_Dig_18_Sts_IN_DIG_DIAG_002400  DataType=uint16  Init=0  Slope=1  Bias=0  DataSize=1  fpDataType=uint16  BlockIOType=Outport  DeviceType=0
  out_OUT_FMSCAN.Tx_Dig.In_Dig_18_Sts.IN_DIG_Val : KIBES_Signal/KIBES_Signal  MBDS_LibraryBlock=on  DatabaseKey=2401  SignalName=OUT_FMSCAN.Tx_Dig.In_Dig_18_Sts.IN_DIG_Val  SymbolName=OUT_FMSCAN_Tx_Dig_In_Dig_18_Sts_IN_DIG_Val_002401  DataType=boolean  Init=0  Slope=1  Bias=0  DataSize=1  fpDataType=boolean  BlockIOType=Outport  DeviceType=0
  out_OUT_FMSCAN.Tx_Dig.In_Dig_18_Sts.MessageEnable : KIBES_Signal/KIBES_Signal  MBDS_LibraryBlock=on  DatabaseKey=2427  SignalName=OUT_FMSCAN.Tx_Dig.In_Dig_18_Sts.MessageEnable  SymbolName=OUT_FMSCAN_Tx_Dig_In_Dig_18_Sts_MessageEnable_002427  DataType=boolean  Init=0  Slope=1  Bias=0  DataSize=1  fpDataType=boolean  BlockIOType=Outport  DeviceType=0
  out_OUT_FMSCAN.Tx_Dig.In_Dig_19_Sts.IN_DIG_DIAG : KIBES_Signal/KIBES_Signal  MBDS_LibraryBlock=on  DatabaseKey=2402  SignalName=OUT_FMSCAN.Tx_Dig.In_Dig_19_Sts.IN_DIG_DIAG  SymbolName=OUT_FMSCAN_Tx_Dig_In_Dig_19_Sts_IN_DIG_DIAG_002402  DataType=uint16  Init=0  Slope=1  Bias=0  DataSize=1  fpDataType=uint16  BlockIOType=Outport  DeviceType=0
  out_OUT_FMSCAN.Tx_Dig.In_Dig_19_Sts.IN_DIG_Val : KIBES_Signal/KIBES_Signal  MBDS_LibraryBlock=on  DatabaseKey=2403  SignalName=OUT_FMSCAN.Tx_Dig.In_Dig_19_Sts.IN_DIG_Val  SymbolName=OUT_FMSCAN_Tx_Dig_In_Dig_19_Sts_IN_DIG_Val_002403  DataType=boolean  Init=0  Slope=1  Bias=0  DataSize=1  fpDataType=boolean  BlockIOType=Outport  DeviceType=0
  out_OUT_FMSCAN.Tx_Dig.In_Dig_19_Sts.MessageEnable : KIBES_Signal/KIBES_Signal  MBDS_LibraryBlock=on  DatabaseKey=2428  SignalName=OUT_FMSCAN.Tx_Dig.In_Dig_19_Sts.MessageEnable  SymbolName=OUT_FMSCAN_Tx_Dig_In_Dig_19_Sts_MessageEnable_002428  DataType=boolean  Init=0  Slope=1  Bias=0  DataSize=1  fpDataType=boolean  BlockIOType=Outport  DeviceType=0
  out_OUT_FMSCAN.Tx_Dig.In_Dig_20_Sts.IN_DIG_DIAG : KIBES_Signal/KIBES_Signal  MBDS_LibraryBlock=on  DatabaseKey=2404  SignalName=OUT_FMSCAN.Tx_Dig.In_Dig_20_Sts.IN_DIG_DIAG  SymbolName=OUT_FMSCAN_Tx_Dig_In_Dig_20_Sts_IN_DIG_DIAG_002404  DataType=uint16  Init=0  Slope=1  Bias=0  DataSize=1  fpDataType=uint16  BlockIOType=Outport  DeviceType=0
  out_OUT_FMSCAN.Tx_Dig.In_Dig_20_Sts.IN_DIG_Val : KIBES_Signal/KIBES_Signal  MBDS_LibraryBlock=on  DatabaseKey=2405  SignalName=OUT_FMSCAN.Tx_Dig.In_Dig_20_Sts.IN_DIG_Val  SymbolName=OUT_FMSCAN_Tx_Dig_In_Dig_20_Sts_IN_DIG_Val_002405  DataType=boolean  Init=0  Slope=1  Bias=0  DataSize=1  fpDataType=boolean  BlockIOType=Outport  DeviceType=0
  out_OUT_FMSCAN.Tx_Dig.In_Dig_20_Sts.MessageEnable : KIBES_Signal/KIBES_Signal  MBDS_LibraryBlock=on  DatabaseKey=2429  SignalName=OUT_FMSCAN.Tx_Dig.In_Dig_20_Sts.MessageEnable  SymbolName=OUT_FMSCAN_Tx_Dig_In_Dig_20_Sts_MessageEnable_002429  DataType=boolean  Init=0  Slope=1  Bias=0  DataSize=1  fpDataType=boolean  BlockIOType=Outport  DeviceType=0
  out_OUT_FMSCAN.Tx_Dig.In_Dig_21_Sts.IN_DIG_DIAG : KIBES_Signal/KIBES_Signal  MBDS_LibraryBlock=on  DatabaseKey=2406  SignalName=OUT_FMSCAN.Tx_Dig.In_Dig_21_Sts.IN_DIG_DIAG  SymbolName=OUT_FMSCAN_Tx_Dig_In_Dig_21_Sts_IN_DIG_DIAG_002406  DataType=uint16  Init=0  Slope=1  Bias=0  DataSize=1  fpDataType=uint16  BlockIOType=Outport  DeviceType=0
  out_OUT_FMSCAN.Tx_Dig.In_Dig_21_Sts.IN_DIG_Val : KIBES_Signal/KIBES_Signal  MBDS_LibraryBlock=on  DatabaseKey=2407  SignalName=OUT_FMSCAN.Tx_Dig.In_Dig_21_Sts.IN_DIG_Val  SymbolName=OUT_FMSCAN_Tx_Dig_In_Dig_21_Sts_IN_DIG_Val_002407  DataType=boolean  Init=0  Slope=1  Bias=0  DataSize=1  fpDataType=boolean  BlockIOType=Outport  DeviceType=0
  out_OUT_FMSCAN.Tx_Dig.In_Dig_21_Sts.MessageEnable : KIBES_Signal/KIBES_Signal  MBDS_LibraryBlock=on  DatabaseKey=2430  SignalName=OUT_FMSCAN.Tx_Dig.In_Dig_21_Sts.MessageEnable  SymbolName=OUT_FMSCAN_Tx_Dig_In_Dig_21_Sts_MessageEnable_002430  DataType=boolean  Init=0  Slope=1  Bias=0  DataSize=1  fpDataType=boolean  BlockIOType=Outport  DeviceType=0
  out_OUT_FMSCAN.Tx_Dig.In_Dig_22_Sts.IN_DIG_DIAG : KIBES_Signal/KIBES_Signal  MBDS_LibraryBlock=on  DatabaseKey=2408  SignalName=OUT_FMSCAN.Tx_Dig.In_Dig_22_Sts.IN_DIG_DIAG  SymbolName=OUT_FMSCAN_Tx_Dig_In_Dig_22_Sts_IN_DIG_DIAG_002408  DataType=uint16  Init=0  Slope=1  Bias=0  DataSize=1  fpDataType=uint16  BlockIOType=Outport  DeviceType=0
  out_OUT_FMSCAN.Tx_Dig.In_Dig_22_Sts.IN_DIG_Val : KIBES_Signal/KIBES_Signal  MBDS_LibraryBlock=on  DatabaseKey=2409  SignalName=OUT_FMSCAN.Tx_Dig.In_Dig_22_Sts.IN_DIG_Val  SymbolName=OUT_FMSCAN_Tx_Dig_In_Dig_22_Sts_IN_DIG_Val_002409  DataType=boolean  Init=0  Slope=1  Bias=0  DataSize=1  fpDataType=boolean  BlockIOType=Outport  DeviceType=0
  out_OUT_FMSCAN.Tx_Dig.In_Dig_22_Sts.MessageEnable : KIBES_Signal/KIBES_Signal  MBDS_LibraryBlock=on  DatabaseKey=2431  SignalName=OUT_FMSCAN.Tx_Dig.In_Dig_22_Sts.MessageEnable  SymbolName=OUT_FMSCAN_Tx_Dig_In_Dig_22_Sts_MessageEnable_002431  DataType=boolean  Init=0  Slope=1  Bias=0  DataSize=1  fpDataType=boolean  BlockIOType=Outport  DeviceType=0
  tag scope: InDig01=global, InDig02=global, InDig05=global, InDig06=global, InDig07=global, InDig08=global, InDig09=global, InDig10=global
  wires:
  in_DIAG_ACAN.BSG_EXPA.IN_DIG_01_DIAG/1 -> out_OUT_FMSCAN.Tx_Dig.In_Dig_01_Sts.IN_DIG_DIAG/1
  in_DIAG_ACAN.BSG_EXPA.IN_DIG_08_DIAG/1 -> out_OUT_FMSCAN.Tx_Dig.In_Dig_08_Sts.IN_DIG_DIAG/1
  in_DIAG_ACAN.BSG_EXPA.IN_DIG_09_DIAG/1 -> out_OUT_FMSCAN.Tx_Dig.In_Dig_09_Sts.IN_DIG_DIAG/1
  in_IN_ACAN.BSG_EXPA.IN_DIG_09/1 -> out_OUT_FMSCAN.Tx_Dig.In_Dig_09_Sts.IN_DIG_Val/1, [InDig09]
  in_IN_ACAN.BSG_EXPA.IN_DIG_10/1 -> out_OUT_FMSCAN.Tx_Dig.In_Dig_10_Sts.IN_DIG_Val/1, [InDig10]
  in_DIAG_ACAN.BSG_EXPA.IN_DIG_13_DIAG/1 -> out_OUT_FMSCAN.Tx_Dig.In_Dig_13_Sts.IN_DIG_DIAG/1
  in_IN_ACAN.BSG_EXPA.IN_DIG_03/1 -> out_OUT_FMSCAN.Tx_Dig.In_Dig_03_Sts.IN_DIG_Val/1
  in_IN_ACAN.BSG_EXPA.IN_DIG_02/1 -> out_OUT_FMSCAN.Tx_Dig.In_Dig_02_Sts.IN_DIG_Val/1, [InDig02]
  in_IN_ACAN.BSG_EXPA.IN_DIG_01/1 -> out_OUT_FMSCAN.Tx_Dig.In_Dig_01_Sts.IN_DIG_Val/1, [InDig01]
  in_IN_ACAN.BSG_EXPA.IN_DIG_21/1 -> out_OUT_FMSCAN.Tx_Dig.In_Dig_21_Sts.IN_DIG_Val/1
  in_IN_ACAN.BSG_EXPA.IN_DIG_16/1 -> out_OUT_FMSCAN.Tx_Dig.In_Dig_16_Sts.IN_DIG_Val/1
  in_IN_ACAN.BSG_EXPA.IN_DIG_14/1 -> out_OUT_FMSCAN.Tx_Dig.In_Dig_14_Sts.IN_DIG_Val/1
  in_DIAG_ACAN.BSG_EXPA.IN_DIG_02_DIAG/1 -> out_OUT_FMSCAN.Tx_Dig.In_Dig_02_Sts.IN_DIG_DIAG/1
  in_IN_ACAN.BSG_EXPA.IN_DIG_18/1 -> out_OUT_FMSCAN.Tx_Dig.In_Dig_18_Sts.IN_DIG_Val/1
  in_IN_ACAN.BSG_EXPA.IN_DIG_11/1 -> out_OUT_FMSCAN.Tx_Dig.In_Dig_11_Sts.IN_DIG_Val/1
  in_DIAG_ACAN.BSG_EXPA.IN_DIG_22_DIAG/1 -> out_OUT_FMSCAN.Tx_Dig.In_Dig_22_Sts.IN_DIG_DIAG/1
  in_DIAG_ACAN.BSG_EXPA.IN_DIG_21_DIAG/1 -> out_OUT_FMSCAN.Tx_Dig.In_Dig_21_Sts.IN_DIG_DIAG/1
  in_DIAG_ACAN.BSG_EXPA.IN_DIG_20_DIAG/1 -> out_OUT_FMSCAN.Tx_Dig.In_Dig_20_Sts.IN_DIG_DIAG/1
  in_DIAG_ACAN.BSG_EXPA.IN_DIG_16_DIAG/1 -> out_OUT_FMSCAN.Tx_Dig.In_Dig_16_Sts.IN_DIG_DIAG/1
  in_IN_ACAN.BSG_EXPA.IN_DIG_13/1 -> out_OUT_FMSCAN.Tx_Dig.In_Dig_13_Sts.IN_DIG_Val/1
  in_DIAG_ACAN.BSG_EXPA.IN_DIG_14_DIAG/1 -> out_OUT_FMSCAN.Tx_Dig.In_Dig_14_Sts.IN_DIG_DIAG/1
  in_DIAG_ACAN.BSG_EXPA.IN_DIG_12_DIAG/1 -> out_OUT_FMSCAN.Tx_Dig.In_Dig_12_Sts.IN_DIG_DIAG/1
  in_IN_ACAN.BSG_EXPA.IN_DIG_20/1 -> out_OUT_FMSCAN.Tx_Dig.In_Dig_20_Sts.IN_DIG_Val/1
  in_IN_ACAN.BSG_EXPA.IN_DIG_12/1 -> out_OUT_FMSCAN.Tx_Dig.In_Dig_12_Sts.IN_DIG_Val/1
  in_DIAG_ACAN.BSG_EXPA.IN_DIG_05_DIAG/1 -> out_OUT_FMSCAN.Tx_Dig.In_Dig_05_Sts.IN_DIG_DIAG/1
  in_DIAG_ACAN.BSG_EXPA.IN_DIG_15_DIAG/1 -> out_OUT_FMSCAN.Tx_Dig.In_Dig_15_Sts.IN_DIG_DIAG/1
  in_DIAG_ACAN.BSG_EXPA.IN_DIG_04_DIAG/1 -> out_OUT_FMSCAN.Tx_Dig.In_Dig_04_Sts.IN_DIG_DIAG/1
  in_DIAG_ACAN.BSG_EXPA.IN_DIG_03_DIAG/1 -> out_OUT_FMSCAN.Tx_Dig.In_Dig_03_Sts.IN_DIG_DIAG/1
  in_DIAG_ACAN.BSG_EXPA.IN_DIG_10_DIAG/1 -> out_OUT_FMSCAN.Tx_Dig.In_Dig_10_Sts.IN_DIG_DIAG/1
  in_IN_ACAN.BSG_EXPA.IN_DIG_17/1 -> out_OUT_FMSCAN.Tx_Dig.In_Dig_17_Sts.IN_DIG_Val/1
  in_IN_ACAN.BSG_EXPA.IN_DIG_04/1 -> out_OUT_FMSCAN.Tx_Dig.In_Dig_04_Sts.IN_DIG_Val/1
  in_DIAG_ACAN.BSG_EXPA.IN_DIG_19_DIAG/1 -> out_OUT_FMSCAN.Tx_Dig.In_Dig_19_Sts.IN_DIG_DIAG/1
  in_DIAG_ACAN.BSG_EXPA.IN_DIG_11_DIAG/1 -> out_OUT_FMSCAN.Tx_Dig.In_Dig_11_Sts.IN_DIG_DIAG/1
  in_DIAG_ACAN.BSG_EXPA.IN_DIG_07_DIAG/1 -> out_OUT_FMSCAN.Tx_Dig.In_Dig_07_Sts.IN_DIG_DIAG/1
  in_IN_ACAN.BSG_EXPA.IN_DIG_15/1 -> out_OUT_FMSCAN.Tx_Dig.In_Dig_15_Sts.IN_DIG_Val/1
  in_IN_ACAN.BSG_EXPA.IN_DIG_08/1 -> out_OUT_FMSCAN.Tx_Dig.In_Dig_08_Sts.IN_DIG_Val/1, [InDig08]
  in_IN_ACAN.BSG_EXPA.IN_DIG_22/1 -> out_OUT_FMSCAN.Tx_Dig.In_Dig_22_Sts.IN_DIG_Val/1
  in_IN_ACAN.BSG_EXPA.IN_DIG_19/1 -> out_OUT_FMSCAN.Tx_Dig.In_Dig_19_Sts.IN_DIG_Val/1
  in_DIAG_ACAN.BSG_EXPA.IN_DIG_06_DIAG/1 -> out_OUT_FMSCAN.Tx_Dig.In_Dig_06_Sts.IN_DIG_DIAG/1
  in_DIAG_ACAN.BSG_EXPA.IN_DIG_18_DIAG/1 -> out_OUT_FMSCAN.Tx_Dig.In_Dig_18_Sts.IN_DIG_DIAG/1
  in_IN_ACAN.BSG_EXPA.IN_DIG_07/1 -> out_OUT_FMSCAN.Tx_Dig.In_Dig_07_Sts.IN_DIG_Val/1, [InDig07]
  bo_SendEnable/1 -> out_OUT_FMSCAN.Tx_Dig.In_Dig_21_Sts.MessageEnable/1, out_OUT_FMSCAN.Tx_Dig.In_Dig_22_Sts.MessageEnable/1, out_OUT_FMSCAN.Tx_Dig.In_Dig_20_Sts.MessageEnable/1, out_OUT_FMSCAN.Tx_Dig.In_Dig_19_Sts.MessageEnable/1, out_OUT_FMSCAN.Tx_Dig.In_Dig_18_Sts.MessageEnable/1, out_OUT_FMSCAN.Tx_Dig.In_Dig_17_Sts.MessageEnable/1, out_OUT_FMSCAN.Tx_Dig.In_Dig_16_Sts.MessageEnable/1, out_OUT_FMSCAN.Tx_Dig.In_Dig_15_Sts.MessageEnable/1, out_OUT_FMSCAN.Tx_Dig.In_Dig_14_Sts.MessageEnable/1, out_OUT_FMSCAN.Tx_Dig.In_Dig_13_Sts.MessageEnable/1, out_OUT_FMSCAN.Tx_Dig.In_Dig_12_Sts.MessageEnable/1, out_OUT_FMSCAN.Tx_Dig.In_Dig_11_Sts.MessageEnable/1, out_OUT_FMSCAN.Tx_Dig.In_Dig_10_Sts.MessageEnable/1, out_OUT_FMSCAN.Tx_Dig.In_Dig_09_Sts.MessageEnable/1, out_OUT_FMSCAN.Tx_Dig.In_Dig_08_Sts.MessageEnable/1, out_OUT_FMSCAN.Tx_Dig.In_Dig_07_Sts.MessageEnable/1, out_OUT_FMSCAN.Tx_Dig.In_Dig_06_Sts.MessageEnable/1, out_OUT_FMSCAN.Tx_Dig.In_Dig_05_Sts.MessageEnable/1, out_OUT_FMSCAN.Tx_Dig.In_Dig_04_Sts.MessageEnable/1, out_OUT_FMSCAN.Tx_Dig.In_Dig_03_Sts.MessageEnable/1, out_OUT_FMSCAN.Tx_Dig.In_Dig_02_Sts.MessageEnable/1, out_OUT_FMSCAN.Tx_Dig.In_Dig_01_Sts.MessageEnable/1
  in_IN_ACAN.BSG_EXPA.IN_DIG_05/1 -> out_OUT_FMSCAN.Tx_Dig.In_Dig_05_Sts.IN_DIG_Val/1, [InDig05]
  in_IN_ACAN.BSG_EXPA.IN_DIG_06/1 -> out_OUT_FMSCAN.Tx_Dig.In_Dig_06_Sts.IN_DIG_Val/1, [InDig06]
  in_DIAG_ACAN.BSG_EXPA.IN_DIG_17_DIAG/1 -> out_OUT_FMSCAN.Tx_Dig.In_Dig_17_Sts.IN_DIG_DIAG/1

== system MBDS_Subsystems/SUB_ExpIOControl/FrequencyInput ==
  bo_SendEnable : Inport
  in_IN_ACAN.BSG_EXPA.Frequency : KIBES_Signal/KIBES_Signal  MBDS_LibraryBlock=on  DatabaseKey=2296  SignalName=IN_ACAN.BSG_EXPA.Frequency  SymbolName=IN_ACAN_BSG_EXPA_Frequency_002296  DataType=uint16  Init=0  Slope=1  Bias=0  DataSize=1  fpDataType=uint16  BlockIOType=Inport  DeviceType=0
  out_OUT_FMSCAN.Tx_Freq.In_Freq_01_Sts.MessageEnable : KIBES_Signal/KIBES_Signal  MBDS_LibraryBlock=on  DatabaseKey=2638  SignalName=OUT_FMSCAN.Tx_Freq.In_Freq_01_Sts.MessageEnable  SymbolName=OUT_FMSCAN_Tx_Freq_In_Freq_01_Sts_MessageEnable_002638  DataType=boolean  Init=0  Slope=1  Bias=0  DataSize=1  fpDataType=boolean  BlockIOType=Outport  DeviceType=0
  out_OUT_FMSCAN.Tx_Freq.In_Freq_01_Sts.Value : KIBES_Signal/KIBES_Signal  MBDS_LibraryBlock=on  DatabaseKey=2637  SignalName=OUT_FMSCAN.Tx_Freq.In_Freq_01_Sts.Value  SymbolName=OUT_FMSCAN_Tx_Freq_In_Freq_01_Sts_Value_002637  DataType=uint16  Init=0  Slope=1  Bias=0  DataSize=1  fpDataType=uint16  BlockIOType=Outport  DeviceType=0
  wires:
  bo_SendEnable/1 -> out_OUT_FMSCAN.Tx_Freq.In_Freq_01_Sts.MessageEnable/1
  in_IN_ACAN.BSG_EXPA.Frequency/1 -> out_OUT_FMSCAN.Tx_Freq.In_Freq_01_Sts.Value/1
